simulink library "simulink"  (Simulink 7.6)
settings: Solver=ode45  SolverMode=SingleTasking  StartTime=0.0  StopTime=10.0  RelTol=1e-3
PostLoadFcn:
  | setsysloc(bdroot)
undefined symbols (not defined in the file or in its folder): DiscIntNeverNeededParam, Floor, getdatatypespecs, NumBits1, NumBits2, sfunxy, sigbuilder_block, slcm, SlDemoSign, Slope1, Slope2
libraries: simulink x40, sl_helperblocks x2, eml_lib x1
(part 3 of 5)

== system simulink/Model-Wide Utilities ==
  note: Linearization of Running Models
  note: Documentation
  note: Modeling Guides
  Block Support Table : Subsystem
      settings: OpenFcn=showblockdatatypetable
      mask Type: Block Support Table
      mask Description: Double-clicking the block will launch the Simulink Block Data Type Support Table.
      mask Display: disp('Block Support\nTable');
  DocBlock : Subsystem  mask(DocBlock){ECoderFlag=, DocumentType=Text}
      mask prompts: ECoderFlag "RTW Embedded Coder Flag"; DocumentType "Document Type"
      mask help: Use this block to save long descriptive text with the model. Double-clicking the block will open an editor.
      settings: DeleteFcn=docblock('close_document',gcb);  PreSaveFcn=docblock('save_document',gcb);  OpenFcn=docblock('edit_document',gcb);
      mask StyleString: edit,popup(Text|RTF|HTML)
      mask Display:
      | plot([.8 0 0 1 1 .8 .8 1],[1 1 0 0 .8 1 .8 .8]);
      | text(.5,.6,'DOC','horizontalalignment','center');
      | text(.95,.05,get_param(gcb,'DocumentType'),'verticalalignment','bottom','horizontalalignment','right');
  Model Info : Subsystem  LoadFcn=slcm LoadBlock;  InitFcn=slcm('UpdateAllCMBlocksInThisModelInit')  mask(CMBlock){InitialSaveTempField=, InitialBlockCM=none, BlockCM=none, Frame=on, SaveTempField=, DisplayStringWithTags=Model Info, MaskDisplayString=Model Info, HorizontalTextAlignment=Center, LeftAlignmentValue=0.5, SourceBlockDiagram=simulink, TagMaxNumber=20, CMTag1=, CMTag2=, CMTag3=, CMTag4=, CMTag5=, CMTag6=, CMTag7=, CMTag8=, CMTag9=, CMTag10=, CMTag11=, CMTag12=, CMTag13=, CMTag14=, CMTag15=, CMTag16=, CMTag17=, CMTag18=, CMTag19=, CMTag20=}
      mask help: This block allows revision control information to be displayed within the model.
      settings: CopyFcn=slcm CopyBlock;  DeleteFcn=slcm Cancel;  PostSaveFcn=slcm('UpdateAllCMBlocksInThisModel')  NameChangeFcn=slcm Rename;  OpenFcn=slcm
      mask Display: text(str2num(LeftAlignmentValue), 0.5, MaskDisplayString, 'HorizontalAlignment', HorizontalTextAlignment)
  Timed-Based Linearization : Subsystem  mask(Timed Linearization){LinearizationTime=1, SampleTime=0}
      mask prompts: LinearizationTime "Linearization time:"; SampleTime "Sample time (of linearized model):"
      mask help: Generate linear models in the base workspace at specific times.
      mask init:
      | name_  = linsetup;
      mask Help: This block calls LINMOD or DLINMOD to create a linear model for the system when the simulation clock reaches the time specified by the LinearizationTime parameter.  No trimming is performed.  The linear model is stored in the base workspace as a structure, along with information about the operating point at which the snapshot was taken.  Multiple snapshots are appended to form an array of structures.
      mask Display: disp(['T=' mat2str(double(LinearizationTime))])
  Trigger-Based Linearization : Subsystem  TreatAsAtomicUnit=on  mask(Triggered Linearization){TriggerType=rising, SampleTime=0}
      mask prompts: TriggerType "Trigger type:"; SampleTime "Sample time (of linearized model):"
      mask help: Generates linear models in the base workspace when triggered.
      mask init:
      | name_ = linsetup;
      | set_param([ gcb '/Trigger'],'TriggerType',TriggerType);
      mask Help: When triggered, this block calls LINMOD or DLINMOD to create a linear model for the system at the current operating point.  No trimming is performed.   The linear model is stored in the base workspace as a structure, along with information about the operating point at which the snapshot was taken.  Multiple snapshots are appended to form an array of structures.
      mask StyleString: popup(rising|falling|either|function-call),edit

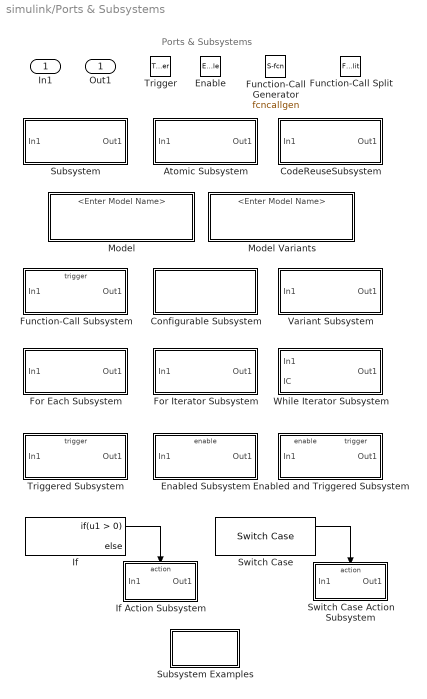
== system simulink/Ports & Subsystems ==
  note: Ports & Subsystems
  In1 : Inport
  Enable : EnablePort
  Trigger : TriggerPort
  Atomic Subsystem : Subsystem  TreatAsAtomicUnit=on
      settings: CopyFcn=set_param(gcbh,'LinkStatus','none'); set_param(gcbh,'Mask','off'); set_param(gcbh,'MaskType',''); set_param(gcbh,'MaskDescription',''); set_param(gcbh,'OpenFcn',''); set_param(gcbh,'CopyFcn','')  OpenFcn=open_system(gcbh,'force')
      mask Type: Atomic Subsystem
      mask Description: A subsystem block template containing an inport and outport block.
  CodeReuseSubsystem : Subsystem  TreatAsAtomicUnit=on
      settings: CopyFcn=set_param(gcbh,'LinkStatus','none'); set_param(gcbh,'Mask','off'); set_param(gcbh,'MaskType',''); set_param(gcbh,'MaskDescription',''); set_param(gcbh,'OpenFcn',''); set_param(gcbh,'CopyFcn','')  OpenFcn=open_system(gcb,'force')  RTWFcnNameOpts=Use subsystem name  RTWFileNameOpts=Use function name
      mask Type: Code Reuse Subsystem
      mask Description: A subsystem block template containing an inport and outport block.
  Configurable Subsystem : Subsystem
      settings: TemplateBlock=master
  Enabled Subsystem : Subsystem  TreatAsAtomicUnit=on
      settings: CopyFcn=set_param(gcbh,'LinkStatus','none'); set_param(gcbh,'Mask','off'); set_param(gcbh,'MaskType',''); set_param(gcbh,'MaskDescription',''); set_param(gcbh,'OpenFcn',''); set_param(gcbh,'CopyFcn','')  OpenFcn=open_system(gcbh,'force')
      mask Type: Enabled Subsystem
      mask Description: A subsystem block template containing an enable port, inport and outport block.
  Enabled and Triggered Subsystem : Subsystem  TreatAsAtomicUnit=on
      settings: CopyFcn=set_param(gcbh,'LinkStatus','none'); set_param(gcbh,'Mask','off'); set_param(gcbh,'MaskType',''); set_param(gcbh,'MaskDescription',''); set_param(gcbh,'OpenFcn',''); set_param(gcbh,'CopyFcn','')  OpenFcn=open_system(gcbh,'force')
      mask Type: Enabled And Triggered Subsystem
      mask Description: A subsystem block template containing an enable port, trigger port, inport and outport block.
  For Each Subsystem : Subsystem  TreatAsAtomicUnit=on
      settings: CopyFcn=set_param(gcbh,'LinkStatus','none'); set_param(gcbh,'Mask','off'); set_param(gcbh,'MaskType',''); set_param(gcbh,'MaskDescription',''); set_param(gcbh,'OpenFcn',''); set_param(gcbh,'CopyFcn','')  OpenFcn=open_system(gcbh,'force')
      mask Type: For Each Subsystem
      mask Description: A subsystem block template containing a for each, inport and outport block.
  For Iterator Subsystem : Subsystem  TreatAsAtomicUnit=on
      settings: CopyFcn=set_param(gcbh,'LinkStatus','none'); set_param(gcbh,'Mask','off'); set_param(gcbh,'MaskType',''); set_param(gcbh,'MaskDescription',''); set_param(gcbh,'OpenFcn',''); set_param(gcbh,'CopyFcn','')  OpenFcn=open_system(gcbh,'force')
      mask Type: For Iterator Subsystem
      mask Description: A subsystem block template containing a for iterator, inport and outport block.
  Function-Call Generator : S-Function  FunctionName=fcncallgen  Parameters=sample_time,numberOfIterations  EnableBusSupport=off  mask(Function-Call Generator){sample_time=1, numberOfIterations=1}
      mask prompts: sample_time "Sample time:"; numberOfIterations "Number of iterations:"
      mask help:
      | This block implements an iterator operation. On each time-step as defined by the sample time field, this block will execute the function-call subsystem(s) that it drives for the specified number of iterations.
      |
      | Demux the block's output to execute multiple function-call subsystems in a prescribed order.  The system connected to first demux port is executed first, the system connected to second demux port is executed second, and so on.
      mask init:
      | if ~isempty(numberOfIterations) & length(numberOfIterations) == 1 & (numberOfIterations > 1),
      | str=sprintf('iterate I = 1:%d',numberOfIterations);
      | else, str = 'f()';
      | end;
      mask Help: This block executes a function-call subsystem at the rate specified by the sample time and a specified number of times.
      mask Display: disp(str)
  Function-Call Split : FunctionCallSplit
      settings: CopyFcn=set_param(gcbh,'ShowName','off','CopyFcn','')
  Function-Call Subsystem : Subsystem  TreatAsAtomicUnit=on
      settings: CopyFcn=set_param(gcbh,'LinkStatus','none'); set_param(gcbh,'Mask','off'); set_param(gcbh,'MaskType',''); set_param(gcbh,'MaskDescription',''); set_param(gcbh,'OpenFcn',''); set_param(gcbh,'CopyFcn','')  OpenFcn=open_system(gcbh,'force')
      mask Type: Function-Call Subsystem
      mask Description: A subsystem block template containing a function-call trigger port, inport and outport block.
  If : If
  If Action Subsystem : Subsystem  TreatAsAtomicUnit=on
      settings: CopyFcn=set_param(gcbh,'LinkStatus','none'); set_param(gcbh,'Mask','off'); set_param(gcbh,'MaskType',''); set_param(gcbh,'MaskDescription',''); set_param(gcbh,'OpenFcn',''); set_param(gcbh,'CopyFcn','')  OpenFcn=open_system(gcbh,'force')
      mask Type: If Action Subsystem
      mask Description: A subsystem block template containing an action port, inport and outport block.
  Model : ModelReference  ModelNameDialog=<Enter Model Name>  SimulationMode=Accelerator
  Model Variants : ModelReference  ModelNameDialog=<Enter Model Name>  SimulationMode=Accelerator  Variant=on
      settings: AttributesFormatString=%<ActiveVariant>
  Subsystem : Subsystem
      settings: CopyFcn=set_param(gcbh,'LinkStatus','none'); set_param(gcbh,'Mask','off'); set_param(gcbh,'MaskType',''); set_param(gcbh,'MaskDescription',''); set_param(gcbh,'OpenFcn',''); set_param(gcbh,'CopyFcn','')  OpenFcn=open_system(gcbh,'force')
      mask Type: Virtual Subsystem
      mask Description: A subsystem block template containing an inport and outport block.
  Subsystem Examples : Subsystem
      settings: OpenFcn=open_system('sl_subsys_semantics','force')
      mask Type: Subsystem Examples
      mask Description: These are examples of how to use the different types of subsystems.
      mask Display: disp('Subsystem\nExamples')
  Switch Case : SwitchCase
  Switch Case Action Subsystem : Subsystem  TreatAsAtomicUnit=on
      settings: CopyFcn=set_param(gcbh,'LinkStatus','none'); set_param(gcbh,'Mask','off'); set_param(gcbh,'MaskType',''); set_param(gcbh,'MaskDescription',''); set_param(gcbh,'OpenFcn',''); set_param(gcbh,'CopyFcn','')  OpenFcn=open_system(gcbh,'force')
      mask Type: Switch Case Action Subsystem
      mask Description: A subsystem block template containing an action port, inport and outport block.
  Triggered Subsystem : Subsystem  TreatAsAtomicUnit=on
      settings: CopyFcn=set_param(gcbh,'LinkStatus','none'); set_param(gcbh,'Mask','off'); set_param(gcbh,'MaskType',''); set_param(gcbh,'MaskDescription',''); set_param(gcbh,'OpenFcn',''); set_param(gcbh,'CopyFcn','')  OpenFcn=open_system(gcbh,'force')
      mask Type: Triggered Subsystem
      mask Description: A subsystem block template containing a trigger port, inport and outport block.
  Variant Subsystem : Subsystem  Variant=on
      settings: CopyFcn=set_param(gcbh,'LinkStatus','none'); set_param(gcbh,'Mask','off'); set_param(gcbh,'MaskType',''); set_param(gcbh,'MaskDescription',''); set_param(gcbh,'OpenFcn',''); set_param(gcbh,'CopyFcn','')
      mask Type: Variant Subsystem
      mask Description: A Variant Subsystem template containing an inport and outport block
  While Iterator Subsystem : Subsystem  TreatAsAtomicUnit=on
      settings: CopyFcn=set_param(gcbh,'LinkStatus','none'); set_param(gcbh,'Mask','off'); set_param(gcbh,'MaskType',''); set_param(gcbh,'MaskDescription',''); set_param(gcbh,'OpenFcn',''); set_param(gcbh,'CopyFcn','')  OpenFcn=open_system(gcbh,'force')
      mask Type: While Iterator Subsystem
      mask Description: A subsystem block template containing a while iterator, inport and outport block.
  Out1 : Outport
  wires:
  If/1 -> If Action Subsystem/Action
  Switch Case/1 -> Switch Case Action Subsystem/Action

== system simulink/Signal Attributes ==
  note: Signal Attribute Manipulation
  note: Signal Attribute Detection
  Bus to Vector : BusToVector
  Data Type Conversion Inherited : Subsystem  mask(Conversion Inherited){ConvertRealWorld=Real World Value, RndMeth=Floor, DoSatur=off}
      mask prompts: ConvertRealWorld "Input and Output to have equal:"; RndMeth "Integer rounding mode:"; DoSatur "Saturate to max or min when overflows occur"
      mask help:
      | Convert the second input to the data type and scaling of the first input.
      |
      | The conversion has two possible goals.  One goal is to have the Real World Values of the input and the output be equal.  The other goal is to have the Stored Integer Values of the input and the output be equal.  Overflows and quantization errors can prevent the goal from being fully achieved.
      mask init:
      | rndMethCell = {'Ceiling','Convergent','Floor','Nearest','Round','Simplest','Zero'};
      | onOffCell = {'off','on'};
      | RWVvsSICell = { 'Real World Value','Stored Integer'};
      | set_param([gcb,'/Conversion'],'RndMeth',rndMethCell{RndMeth},...
      |                                 'DoSatur',onOffCell{DoSatur+1},...
      |                                 'ConvertRealWorld',RWVvsSICell{ConvertRealWorld});
      mask StyleString: popup(Real World Value|Stored Integer),popup(Ceiling|Convergent|Floor|Nearest|Round|Simplest|Zero),checkbox
      mask Display:
      | port_label('Input',2,'u');
      | port_label('Output',1,'y');
      | disp('Convert')
  Data Type Duplicate : DataTypeDuplicate
  Data Type Propagation : S-Function  FunctionName=sfix_dtprop  Parameters=14,PropDataTypeMode,(getdatatypespecs(PropDataType,PropScaling,DblOver,0, 0, PropDataTypeMode, PropScalingMode)),IfRefDouble,IfRefSingle,IsSigned,NumBitsBase,NumBitsMult,NumBitsAdd,(sort(reshape(round(NumBitsAllowFinal), prod(size(NumBitsAllowFinal)),1))),PropScalingMode,ValuesUsedBestPrec,SlopeBase,SlopeMult,SlopeAdd,BiasBase,BiasMult,BiasAdd,DblOver  EnableBusSupport=off  mask(Data Type Propagation){PropDataTypeMode=Inherit via propagation rule, PropDataType=fixdt(1, 16), IfRefDouble=double, IfRefSingle=single, IsSigned=IsSigned1 or IsSigned2, NumBitsBase=max([NumBits1 NumBits2]), NumBitsMult=1, NumBitsAdd=0, NumBitsAllowFinal=1:128, PropScalingMode=Inherit via propagation rule, PropScaling=2^-10, ValuesUsedBestPrec=[5 -7], SlopeBase=min([Slope1 Slope2]), SlopeMult=1, SlopeAdd=0, BiasBase=Bias1, BiasMult=1, BiasAdd=0}
      mask prompts: PropDataTypeMode "1. Propagated data type:"; PropDataType "1.1. Propagated data type (e.g. fixdt(1, 16), fixdt('single')):"; IfRefDouble "1.1. If any reference input is double, output is:"; IfRefSingle "1.2. If any reference input is single, output is:"; IsSigned "1.3. Is-Signed:"; NumBitsBase "1.4.1. Number-of-Bits: Base"; NumBitsMult "1.4.2. Number-of-Bits: Multiplicative adjustment"; NumBitsAdd "1.4.3. Number-of-Bits: Additive adjustment"; NumBitsAllowFinal "1.4.4. Number-of-Bits: Allowable final values"; PropScalingMode "2. Propagated scaling:"; PropScaling "2.1. Propagated scaling (Slope, e.g. 2^-9 or [Slope Bias], e.g. [1.25 3]):"; ValuesUsedBestPrec "2.1. Values used to determine best precision scaling."; SlopeBase "2.1.1. Slope: Base"; SlopeMult "2.1.2. Slope: Multiplicative adjustment"; SlopeAdd "2.1.3. Slope: Additive adjustment"; BiasBase "2.2.1. Bias: Base"; BiasMult "2.2.2. Bias: Multiplicative adjustment:"; BiasAdd "2.2.3. Bias: Additive adjustment:"
      mask help:
      | Set the Data Type and Scaling of the propagated signal based on information from the reference signals.
      | Notes:
      | 1) Items closer to the top of the dialog have higher priority/precedence.
      | a) Reference inputs of type double have priority over all others.
      | b) Singles have priority over integer and fixed point data types.
      | c) Multiplicative adjustments are carried out before additive adjustments.
      | d) Number-of-Bits is determined before the precision or positive-range is inherited from the reference signals.
      | 2) PosRange is one bit higher than the exact maximum positive range of the signal.
      | 3) The computed Number-of-Bits is promoted to the smallest allowable value that is greater than or equal.  If none exists, then error.
      mask init:
      | DblOver = 0;
      mask StyleString: popup(Specify via dialog|Inherit via propagation rule),edit,popup(double|single),popup(double|single),popup(IsSigned1|IsSigned2|IsSigned1 or IsSigned2|TRUE|FALSE),popup(NumBits1|NumBits2|max([NumBits1 NumBits2])|min([NumBits1 NumBits2])|NumBits1+NumBits2),edit,edit,edit,popup(Specify via dialog|Inherit via propagation rule|Obtain via best precision),edit,edit,popup(Slope1|Slope2|max([Slope1 Slope2])|min([Slope1 Slope2])|Slope1*Slope2|Slope1/Slope2|PosRange1|PosRange2|max([PosRange1 PosRange2])|min([PosRange1 PosRange2])|PosRange1*PosRange2|PosRange1/PosRange2),edit,edit,popup(Bias1|Bias2|max([Bias1 Bias2])|min([Bias1 Bias2])|Bias1*Bias2|Bias1/Bias2|Bias1+Bias2|Bias1-Bias2),edit,edit
      mask CallbackString: fixptdialog(gcbh)|fixptdialog(gcbh)||||||||fixptdialog(gcbh)||||||||
      mask TabNameString: Propagated type,Propagated type,Propagated type,Propagated type,Propagated type,Propagated type,Propagated type,Propagated type,Propagated type,Propagated scaling,Propagated scaling,Propagated scaling,Propagated scaling,Propagated scaling,Propagated scaling,Propagated scaling,Propagated scaling,Propagated scaling
      mask Display:
      | port_label('Input',1,'Ref1');
      | port_label('Input',2,'Ref2');
      | port_label('Input',3,'Prop');
  Data Type Propagation Examples : Subsystem
      settings: OpenFcn=open_system('fixpt_dtprop','force')
      mask Type: Data Type Propagation Examples
      mask Description: Opens a model containing data type propagation examples.
      mask Display: disp('Data Type\nPropagation\nExamples')
  Data Type Scaling Strip : Subsystem
      mask Type: Scaling Strip
      mask Description: This block strips the scaling off a fixed point signal.  It maps the input data type to the smallest built-in data type that has sufficient bits to hold the input.  The stored Integer Value of the input will be the value of the output.  The output always has nominal scaling (slope = 1.0 and bias = 0.0), so the output does not have a distinction between Real World Value and Stored Integer Value.
      mask Display: fprintf('Scaling\nStrip')
  Data Type Conversion : DataTypeConversion
  IC : InitialCondition
  Probe : Probe  ProbeSignalDimensions=on  ProbeFramedSignal=on
  Rate Transition : RateTransition
  Signal Conversion : SignalConversion  ConversionOutput=Contiguous copy
  Signal Specification : SignalSpecification
  Weighted Sample Time : SampleTimeMath  TsampMathOp=Ts Only
  Width : Width

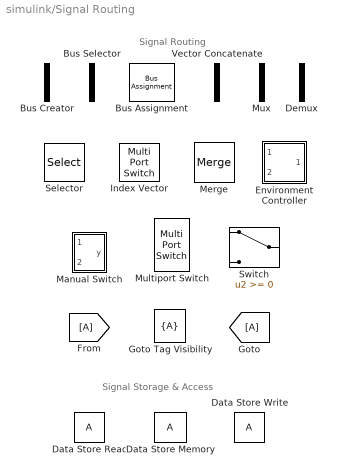
== system simulink/Signal Routing ==
  note: Signal Routing
  note: Signal Storage & Access
  Bus Assignment : BusAssignment
  Bus Creator : BusCreator  Inputs=2
      settings: CopyFcn=set_param(gcbh,'ShowName','off','CopyFcn','')
  Bus Selector : BusSelector  OutputSignals=signal1,signal2
      settings: CopyFcn=set_param(gcbh,'ShowName','off','CopyFcn','')
  Data Store Memory : DataStoreMemory  DataStoreName=A  ReadBeforeWriteMsg=warning  WriteAfterWriteMsg=warning  WriteAfterReadMsg=warning
  Data Store Read : DataStoreRead  DataStoreName=A  SampleTime=-1
  Data Store Write : DataStoreWrite  DataStoreName=A  SampleTime=-1
  Demux : Demux  Outputs=2
      settings: CopyFcn=set_param(gcbh,'ShowName','off','CopyFcn','')
  Environment Controller : Subsystem  mask(Environment Controller){}
      mask help: Output the simulation (Sim) or Real-Time Workshop (RTW) port depending on the current environment. With optimizations enabled, unnecessary blocks leading to the unused port are not executed. Both input signals must be the same width.
      mask init:
      | switch_mode = rtwenvironmentmode(bdroot(gcbh)) || ...
      |     (exist('sldvisactive','file')~=0 && sldvisactive(bdroot(gcbh)));
  Goto Tag Visibility : GotoTagVisibility
  Index Vector : MultiPortSwitch  DataPortOrder=Zero-based contiguous  Inputs=1  zeroidx=on
  Manual Switch : Subsystem  StopFcn=manswitch_config stop;  mask(Manual Switch){sw=1, action=0, varsize=off}
      mask prompts: sw "Current setting:"; varsize "Allow the two inputs to differ in size (Results in variable-size output signal)"
      mask help: Output toggles between two inputs by double-clicking on the block.
      mask init:
      | x=1; y=1;
      | [x,y]=manswitch;
      | manswitch_config;
      settings: OpenFcn=manswitch Open;  ErrorFcn=manswitch
      mask Help: This block implements a manual switch.
      mask Display: plot(x,y)
  Merge : Merge
  Multiport Switch : MultiPortSwitch  zeroidx=off
  Mux : Mux  Inputs=2
      settings: CopyFcn=set_param(gcbh,'ShowName','off','CopyFcn','')
  Selector : Selector  InputPortWidth=3  IndexOptions=Index vector (dialog)  Indices=[1 3]  OutputSizes=1
  Switch : Switch
  Vector Concatenate : Concatenate  Mode=Vector

== system simulink/Sinks ==
  note: Model & Subsystem Outputs
  note: Simulation Control
  note: Data Viewers
  Display : Display
  Floating Scope : Scope
      settings: Floating=on
  Scope : Scope
  Stop Simulation : Stop
  Terminator : Terminator
  To File : ToFile  SaveFormat=Timeseries
  To Workspace : ToWorkspace  VariableName=simout  SampleTime=-1  SaveFormat=Structure
  XY Graph : Subsystem  LoadFcn=sfunxy([],[],[],'LoadBlock')  StartFcn=sfunxy([],[],[],'Start')  StopFcn=sfunxy([],[],[],'Stop')  TreatAsAtomicUnit=on  SimViewingDevice=on  mask(XY scope.){xmin=-1, xmax=1, ymin=-1, ymax=1, st=-1}
      mask prompts: xmin "x-min:"; xmax "x-max:"; ymin "y-min:"; ymax "y-max:"; st "Sample time:"
      mask help: Plots second input (Y) against first input (X) at each time step to create an X-Y plot. Ignores data outside the ranges specified by x-min, x-max, y-min, y-max.
      settings: CopyFcn=sfunxy([],[],[],'CopyBlock')  DeleteFcn=sfunxy([],[],[],'DeleteBlock')  NameChangeFcn=sfunxy([],[],[],'NameChange')
      mask Help: This block can be used to explore limit cycles. Look at the m-file sfunxy.m to see how it works.
      mask Display: plot([.05 .95 .95 .05 .05],[.45 .45 .95 .95 .45], 0.5+cos(0:0.1:2*pi)*0.3,0.7+sin(0:0.1:2*pi)*0.2)
  Out1 : Outport

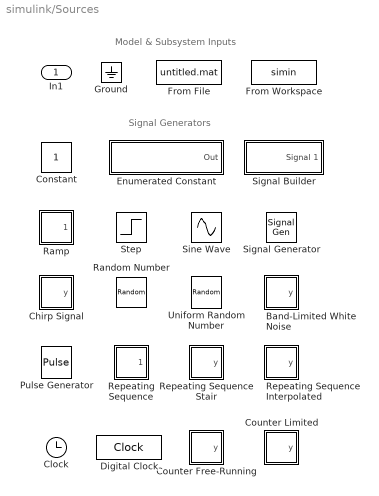
== system simulink/Sources ==
  note: Model & Subsystem Inputs
  note: Signal Generators
  In1 : Inport
  Band-Limited White Noise : Subsystem  mask(Band-Limited White Noise.){Cov=[0.1], Ts=0.1, seed=[23341], VectorParams1D=on}
      mask prompts: Cov "Noise power:"; Ts "Sample time:"; VectorParams1D "Interpret vector parameters as 1-D"
      mask help: The Band-Limited White Noise block generates normally distributed random numbers that are suitable for use in continuous or hybrid systems.
      mask init:
      | if any(Cov < 0),
      | 	error('The ''Noise power'' must be positive. '),
      | end;
      | 
      | r = [-0.4326
      |    -1.6656
      |     0.1253
      |     0.2877
      |    -1.1465
      |     1.1909
      |     1.1892
      |    -0.0376
      |     0.3273
      |     0.1746
      |    -0.1867
      |     0.7258]';
      | 
      | r2 = [r(1),r;r,r(12)]; 
      | t =[1:13;1:13]; 
      | 
      | if any(Ts==-1), 
      | 	error('Sample time (-1) is set to be back-inherited from the block(s) it drives. You should explicitly specify the sample time of the source block. '), 
      | end;
      | set_param([gcb '/White Noise'],'VectorParams1D',VectorParams1D);
      mask Help: Implemented using white noise into Zero-Order Hold block. The seed and power can be vectors of the same length to produce a vector of white noise sources. For faster simulation, set sample time to the highest value possible but in accordance with the fastest dynamics of system.
      mask Display: plot(t(:),r2(:))
  Chirp Signal : Subsystem  mask(chirp){f1=0.1, T=100, f2=1, VectorParams1D=on}
      mask prompts: f1 "Initial frequency (Hz):"; T "Target time (secs):"; f2 "Frequency at target time (Hz):"; VectorParams1D "Interpret vector parameters as 1-D"
      mask help: Output a linear chirp signal (sine wave whose frequency varies linearly with time).
      mask init:
      | blkName = gcb;
      | t=[0:.1:5];
      | set_param([blkName '/targetTime'], 'VectorParams1D', VectorParams1D);
      | set_param([blkName '/initialFreq'], 'VectorParams1D', VectorParams1D);
      | set_param([blkName '/deltaFreq'], 'VectorParams1D', VectorParams1D);
      mask Help: The chirp signal has linearly increasing frequency with time.  This block can be used for spectral analysis of nonlinear systems.
      mask Display: plot(t,sin(t.*t))
  Clock : Clock
      settings: Decimation=10
  Constant : Constant
  Counter Free-Running : Subsystem  mask(Counter Free-Running){NumBits=16, tsamp=-1}
      mask prompts: NumBits "Number of Bits"; tsamp "Sample time:"
      mask help: This block is a free-running counter that overflows back to zero after it has reached the maximum value possible for the specified number of bits. The counter is always initialized to zero. The output is normally an unsigned integer with the specified number of bits.
      mask Display: plot( 0.05+0.9/8*[0 1 1 2 2 3 3 4 4 5 5 6 6 7 7 8 8], 0.3+0.65/3*[0 0 1 1 2 2 3 3 0 0 1 1 2 2 3 3 0] )
  Counter Limited : Subsystem  mask(Counter Limited){uplimit=7, tsamp=-1}
      mask prompts: uplimit "Upper limit:"; tsamp "Sample time:"
      mask help: This block is a counter that wraps back to zero after it has output the specified upper limit. The counter is always initialized to zero. The output is normally an unsigned integer of 8, 16, or 32 bits. The smallest number of bits needed to represent the upper limit is used.
      mask init:
      | nbits = sl('counter_init', uplimit, gcbh);
      mask Display:
      | plot( 0.15+0.8/8*[0 1 1 2 2 3 3 4 4 5 5 6 6 7 7 8 8], 0.3+0.65/3*[0 0 1 1 2 2 3 3 0 0 1 1 2 2 3 3 0] )
      | text(0.05,0.85,'lim')
  Digital Clock : DigitalClock
  Enumerated Constant : Subsystem  DialogController=Simulink.DDGSource  mask(Enumerated Constant){OutDataTypeStr=Enum: SlDemoSign, Value=SlDemoSign.Positive, SampleTime=inf}
      mask prompts: OutDataTypeStr "Output data type:"; SampleTime "Sample time:"
      mask init:
      | % NOTE:
      | % Value is not evaluated to avoid caching an instance
      | % of the MCOS class by the mask infrastructure.
      | 
      | % Get string to use for display purposes
      | enumConstDispStr = Value;
      | if isempty(enumConstDispStr)
      |   enumConstDispStr = '???';
      | end
      | 
      | % Check data type & value
      | enumconst_cb('MaskInit', OutDataTypeStr, slResolve(Value, gcb));
      | 
      | % Set mask parameter values directly on underlying block
      | % and clear mask workspace variables to prevent underlying
      | % blocks from resolving to unevaluated mask variables.
      | set_param([gcb, '/Constant'], ...
      |     'OutDataTypeStr', OutDataTypeStr, ...
      |     'SampleTime',     SampleTime, ...
      |     'Value',          Value);
      | clear OutDataTypeStr SampleTime Value;
      mask Display: disp(enumConstDispStr)
  From Workspace : FromWorkspace  VariableName=simin  SampleTime=0
  From File : FromFile  SampleTime=0
  Ground : Ground
  Pulse Generator : DiscretePulseGenerator  PulseType=Time based  Period=10  PulseWidth=5
  Ramp : Subsystem  mask(Ramp){slope=1, start=0, X0=0, VectorParams1D=on}
      mask prompts: start "Start time:"; X0 "Initial output:"; VectorParams1D "Interpret vector parameters as 1-D"
      mask help: Output a ramp signal starting at the specified time.
      mask init:
      | blkName = gcb;
      | set_param([blkName '/Constant'], 'VectorParams1D',VectorParams1D);
      | set_param([blkName '/Constant1'], 'VectorParams1D',VectorParams1D);
      | set_param([blkName '/Step'], 'VectorParams1D',VectorParams1D);
      mask Display: plot([0:10],[1,1,1,1:8])
  Random Number : RandomNumber  SampleTime=0.1
  Repeating Sequence : Subsystem  mask(Repeating table){rep_seq_t=[0 2], rep_seq_y=[0 2]}
      mask prompts: rep_seq_t "Time values:"; rep_seq_y "Output values:"
      mask help: Output a repeating sequence of numbers specified in a table of time-value pairs. Values of time should be monotonically increasing.
      mask init:
      | if (length(rep_seq_t) ~= length(rep_seq_y)),
      |   error('Length of time vector and output vector must be the same.')
      | end
      | dbl_rep_seq_t = double(rep_seq_t);
      | dbl_rep_seq_y = double(rep_seq_y);
      | period = max(dbl_rep_seq_t) - min(dbl_rep_seq_t);
      | period = str2num(sprintf('%0.5g',period));
      | s = round(length(dbl_rep_seq_t)/50);
      | if s > 0
      |   pts = [1:s:length(dbl_rep_seq_t)];
      |   L   = length(pts);
      | else
      |   L   = length(dbl_rep_seq_t);
      |   pts = [1:L];
      | end
      | 
      | disp_seq_t = reshape(dbl_rep_seq_t(pts),L,1);
      | disp_seq_y = reshape(dbl_rep_seq_y(pts),L,1);
      | disp_period = max(disp_seq_t) - min(disp_seq_t);
      | 
      | disp_seq_t  = repmat(disp_seq_t,1,3) + (ones(L,1)*(disp_period*[0,1,2]));
      | disp_seq_t = [ disp_seq_t(:); disp_seq_t(end) ];
      | disp_seq_y = repmat(disp_seq_y,1,3);
      | disp_seq_y = [ disp_seq_y(:); disp_seq_y(1) ];
      mask Help: Repeats cycle given in table. Time values should be monotonically increasing.
      mask Display: plot( disp_seq_t, disp_seq_y )
  Repeating Sequence Interpolated : Subsystem  mask(Repeating Sequence Interpolated){OutValues=[3 1 4 2 1].', TimeValues=[0 0.1 0.5 0.6 1].', LookUpMeth=Interpolation-Use End Values, tsamp=0.01, OutMin=[], OutMax=[], OutDataTypeStr=double, OutputDataTypeScalingMode=double, OutDataType=fixdt(0,8), OutScaling=2^-10, LockScale=off}
      mask prompts: OutValues "Vector of output values:"; TimeValues "Vector of time values:"; LookUpMeth "Lookup Method:"; tsamp "Sample time:"; OutMin "Output minimum:"; OutMax "Output maximum:"; OutDataTypeStr "Output data type:"; OutputDataTypeScalingMode "Output data type mode:"; OutDataType "Output data type (e.g. fixdt(1, 16), fixdt('single')):"; OutScaling "Output scaling (Slope, e.g. 2^-9 or [Slope Bias], e.g. [1.25 3]):"; LockScale "Lock output data type setting against changes by the fixed-point tools"
      mask help: Discrete time sequence is output, then repeated. Between data points, the specified lookup method is used to determine the output.
      mask init:
      | xx = double(TimeValues);
      | yy = double(OutValues);
      | if min(xx) < 0
      |   error('Negative Time Values are not supported.');
      |   xx = [];
      | elseif min(xx) > 0
      |   xx(2:(end+1)) = xx;
      |   xx(1) = 0;
      |   yy(2:(end+1)) = yy;
      | end
      | if tsamp == -1
      |   tsamp = min(diff(xx));
      | end
      | nn = floor(max(xx)/double(tsamp));
      | 
      | set_param([gcb,'/Lookup'], ...
      |     'LookUpMeth', LookUpMeth);
      mask StyleString: edit,edit,popup(Interpolation-Use End Values|Use Input Nearest|Use Input Below|Use Input Above),edit,min,max,unidt({m=7|8|9||10|5|6|1}{i=Inherit: Inherit via back propagation}{b=double|single|int8|uint8|int16|uint16|int32|uint32}{s=UDTBinaryPointMode|UDTSlopeBiasMode}{g=UDTSignedSign|UDTUnsignedSign}),popup(double|single|int8|uint8|int16|uint16|int32|uint32|Specify via dialog|Inherit via back propagation),edit,edit,checkbox
      mask CallbackString: ||||||fixptdialog(gcbh)|fixptdialog(gcbh)|fixptdialog(gcbh)||
      mask TabNameString: Main,Main,Main,Main,Signal Attributes,Signal Attributes,Signal Attributes,Signal Attributes,Signal Attributes,Signal Attributes,Signal Attributes
      mask Display: plot(fixpt_look1_mask_data(xx,yy,1,LookUpMeth+1),fixpt_look1_mask_data(xx,yy,0,LookUpMeth+1))
  Repeating Sequence Stair : Subsystem  mask(Repeating Sequence Stair){OutValues=[3 1 4 2 1].', tsamp=-1, OutMin=[], OutMax=[], OutDataTypeStr=double, OutputDataTypeScalingMode=double, OutDataType=fixdt(0,8), ConRadixGroup=Best Precision: Vector-wise, OutScaling=2^-12, LockScale=off}
      mask prompts: OutValues "Vector of output values:"; tsamp "Sample time:"; OutMin "Output minimum:"; OutMax "Output maximum:"; OutDataTypeStr "Output data type:"; OutputDataTypeScalingMode "Output data type mode:"; OutDataType "Output data type (e.g. fixdt(1, 16), fixdt('single')):"; ConRadixGroup "Output scaling mode:"; OutScaling "Output scaling (Slope, e.g. 2^-9 or [Slope Bias], e.g. [1.25 3]):"; LockScale "Lock output data type setting against changes by the fixed-point tools"
      mask help: Discrete time sequence is output, then repeated.
      mask init:
      | dim = size(OutValues);
      | if length(dim) > 2 || min(dim) ~= 1
      |   [X, Y] =  generateQuestionMarkIconData;
      | error('Parameter ''output values'' must be a vector or a scalar');
      |   else
      |   nn = length(OutValues)-1;
      |   xx = (0:(nn+1));
      |   yy = double([reshape(OutValues,1,(nn+1)) OutValues(end)]);
      |  X = fixpt_look1_mask_data(xx,yy,1,4);
      |  Y = fixpt_look1_mask_data(xx,yy,0,4);
      |  end
      mask StyleString: edit,edit,min,max,unidt({m=5|6|7|8|9|3|4|1}{i=Inherit: Inherit via back propagation}{b=double|single|int8|uint8|int16|uint16|int32|uint32|boolean}{s=UDTBinaryPointMode|UDTSlopeBiasMode|UDTBestPrecisionMode}{g=UDTSignedSign|UDTUnsignedSign}{u=enum}),popup(double|single|int8|uint8|int16|uint16|int32|uint32|Specify via dialog|Inherit via back propagation),edit,popup(Use specified scaling|Best Precision: Vector-wise),edit,checkbox
      mask CallbackString: ||||fixptdialog(gcbh)|fixptdialog(gcbh)|fixptdialog(gcbh)|fixptdialog(gcbh)||
      mask TabNameString: Main,Main,Signal Attributes,Signal Attributes,Signal Attributes,Signal Attributes,Signal Attributes,Signal Attributes,Signal Attributes,Signal Attributes
      mask Display: plot(X,Y)
  Signal Generator : SignalGenerator
  Signal Builder : Subsystem  Tag=STV Subsys  LoadFcn=sigbuilder_block('load');  StartFcn=sigbuilder_block('start');  StopFcn=sigbuilder_block('stop');  ClipboardFcn=sigbuilder_block('clipboard');  mask(Sigbuilder block){}
      mask help: Create and generate interchangeable groups of signals whose waveforms are piecewise linear.
      mask init:
      | if ~strcmp(get_param(bdroot(gcbh),'SimulationStatus'),'stopped') tuvar = sigbuilder_block('maskInit'); end
      settings: CopyFcn=sigbuilder_block('copy');  DeleteFcn=sigbuilder_block('delete');  ModelCloseFcn=sigbuilder_block('modelClose');  PreSaveFcn=sigbuilder_block('preSave');  NameChangeFcn=sigbuilder_block('namechange');  OpenFcn=sigbuilder_block('open',[437.6 199.2 550.4 400 ]);  CloseFcn=sigbuilder_block('close');
      mask Display: plot(0,0,100,100,[10,10,40,40,10],[80,20,20,80,80],[40,10],[50,50], [40,27,10],[65,72,56],[40,25,25,10],[28,28,43,43]);
  Sine Wave : Sin  SampleTime=0
  Step : Step  SampleTime=0
  Uniform Random Number : UniformRandomNumber  SampleTime=0.1

== system simulink/User-Defined Functions ==
  note: User-defined Functions
  Embedded MATLAB Function : eml_lib/Embedded MATLAB Function  SystemSampleTime=-1
  Fcn : Fcn  Expr=sin(u(1)*exp(2.3*(-u(2))))
  Level-2 MATLAB S-Function : M-S-Function
  MATLAB Fcn : MATLABFcn
  S-Function : S-Function  EnableBusSupport=off
  S-Function Builder : S-Function  EnableBusSupport=off  mask(S-Function Builder){}
      mask help: The S-Function Builder block creates a wrapper C-MEX S-function from your supplied C code with multiple input ports, output ports, and a variable number of scalar, vector, or matrix parameters. The input and output ports can propagate Simulink built-in data types, fixed-point datatypes, complex, frame, 1-D, and 2-D signals. This block also supports discrete and continuous states of type real. You can optionally have the block generate a TLC file to be used with Real-Time Workshop for code generation.
      mask init:
      | val = [[.9  0.75 0.75 1 1 .9 .9 1]',[1 1 0.75 0.75 .9 .9 1 .9]'];
      | sys = get_param(gcbh,'FunctionName');
      settings: CopyFcn=set_param(gcbh,'LinkStatus','none')  OpenFcn=sfunctionwizard(gcbh)
      mask Display:
      | plot(val(:,1),val(:,2))
      | disp(sys)
  S-Function Examples : Subsystem
      settings: OpenFcn=open_system('sfundemos','force')
      mask Type: S-Function Examples
      mask Description: These are examples of how to use the different types of S-Functions.
      mask Display: disp('S-Function\nExamples')
